simulink model "LanderVehicleSimulation"  (R2023a)
settings: Solver=VariableStepAuto  StartTime=0.0  StopTime=15  RelTol=1e-3
values from neighbouring files (symbols this model uses):
  pLander = 10    [LandingRocketWithMPC1.m]
  references = reshape(info.Xopt',(pPlanner+1)*6,1)    [LandingRocketWithMPC1.m]
  u0 = [0;0]    [LandingRocketWithMPC1.m]
  x0 = [-30;60;0;0;0;0]    [LandingRocketWithMPC1.m]
libraries: simulink x1, mpclib x1
settings Model: Creator=The MathWorks, Inc.  LastModifiedBy=The MathWorks, Inc.
settings DebuggingCC: UnconnectedInputMsg=warning  UnconnectedOutputMsg=warning  UnconnectedLineMsg=warning
settings ModelReferenceCC: EnableRefExpFcnMdlSchedulingChecks=on
settings RTWCC: DLArmComputeVersion=19.05

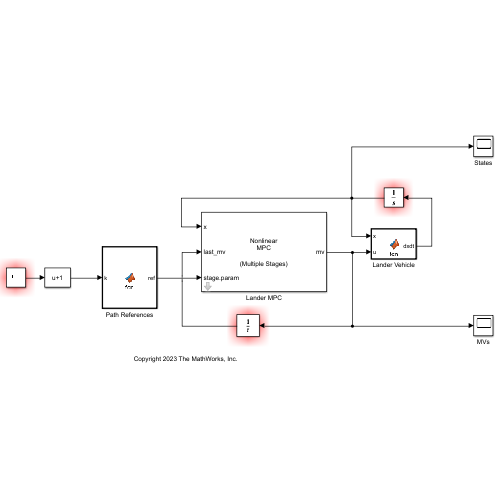
[thumbnail: Simulink's stored preview of the top-level diagram]
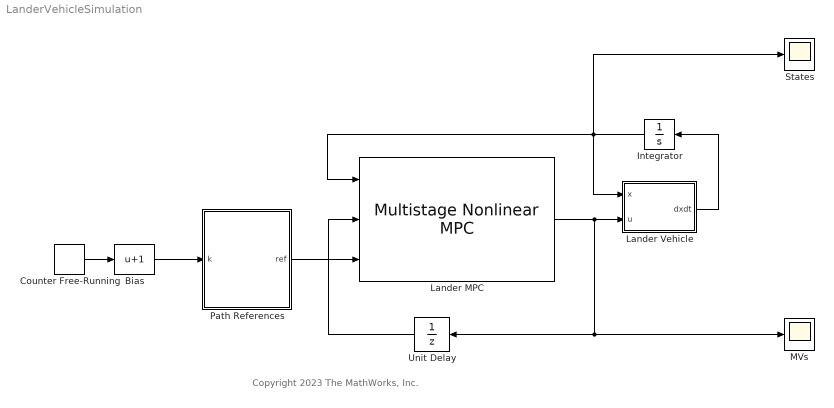
== system LanderVehicleSimulation ==
  note: Copyright 2023 The MathWorks, Inc.
  Bias : Bias  Bias=1  SaturateOnIntegerOverflow=off
  Counter Free-Running : simulink/Sources/Counter Free-Running  NumBits=16  tsamp=Ts
  Integrator : Integrator  InitialCondition=x0
  Lander MPC : mpclib/Multistage Nonlinear MPC  SCDEnableBlockLinearizationSpecification=on  nlmpcobj=lander  UseObjectTs=on  UseMEX=off  md_enabled=off  stateparam_enabled=off  stageparam_enabled=on  cost_enabled=off  mvseq_enabled=off  stateseq_enabled=off  slack_enabled=off  status_enabled=off  mv_min=off  mv_max=off  mvrate_min=off  mvrate_max=off  state_min=off  state_max=off  terminal_state=off  nlp_initialize=off
  Lander Vehicle : MATLAB Function  TreatAsAtomicUnit=on
  MVs : Scope
  Path References : MATLAB Function  TreatAsAtomicUnit=on
  States : Scope
  Unit Delay : UnitDelay  InitialCondition=u0  SampleTime=-1  HasFrameUpgradeWarning=on
  wires:
  Lander MPC/1 -> Unit Delay/1, MVs/1, Lander Vehicle/2(u)
  Lander Vehicle/1(dxdt) -> Integrator/1
  Integrator/1 -> States/1, Lander MPC/1, Lander Vehicle/1(x)
  Unit Delay/1 -> Lander MPC/2
  Path References/1(ref) -> Lander MPC/3
  Counter Free-Running/1 -> Bias/1
  Bias/1 -> Path References/1(k)

== matlab function LanderVehicleSimulation/Lander Vehicle ==
  data: x input; u input; dxdt output
function dxdt = fcn(x,u)
dxdt = LanderVehicleStateFcn(x,u);

== matlab function LanderVehicleSimulation/Path References ==
  data: k input; ref output; references parameter; pLander parameter
function ref = fcn(k,references,pLander)
ref = LanderVehicleReferenceSignal(k,references,pLander);
